simulink model "task2_3"  (R2023a)
settings: Solver=VariableStepAuto  StartTime=0.0  StopTime=10.0  RelTol=1e-3
settings Model: Creator=vasil  LastModifiedBy=vasil

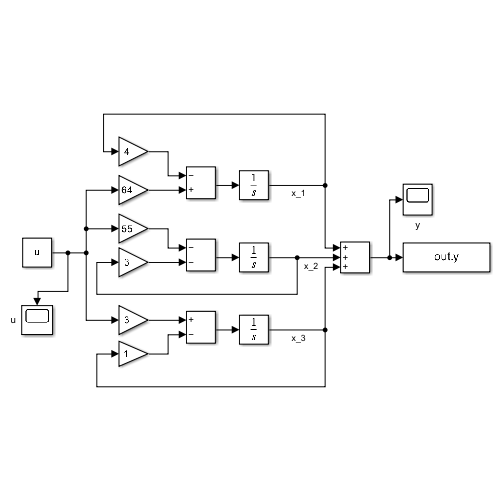
[thumbnail: Simulink's stored preview of the top-level diagram]
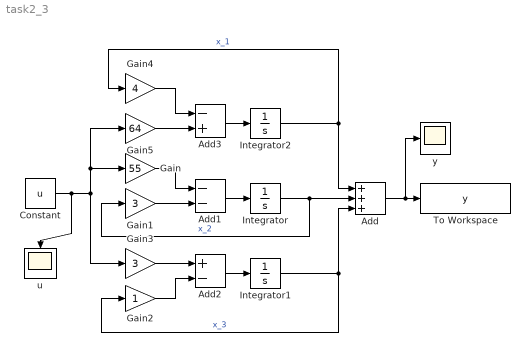
== system task2_3 ==
  Add : Sum  Inputs=+++
  Add1 : Sum  Inputs=--
  Add2 : Sum  Inputs=+-
  Add3 : Sum  Inputs=-+
  Constant : Constant  Value=u
  Gain : Gain  Gain=55
  Gain1 : Gain  Gain=3
  Gain2 : Gain
  Gain3 : Gain  Gain=3
  Gain4 : Gain  Gain=4
  Gain5 : Gain  Gain=64
  Integrator : Integrator
  Integrator1 : Integrator
  Integrator2 : Integrator
  To Workspace : ToWorkspace  VariableName=y  SaveFormat=Timeseries  SampleTime=-1
  u : Scope
  y : Scope
  wires:
  Add/1 -> y/1, To Workspace/1
  Integrator/1 -> Gain1/1, Add/2  "x_2"
  Integrator1/1 -> Gain2/1, Add/3  "x_3"
  Integrator2/1 -> Add/1, Gain4/1  "x_1"
  Add1/1 -> Integrator/1
  Add2/1 -> Integrator1/1
  Add3/1 -> Integrator2/1
  Gain/1 -> Add1/1
  Gain1/1 -> Add1/2
  Constant/1 -> u/1, Gain5/1, Gain/1, Gain3/1
  Gain3/1 -> Add2/1
  Gain2/1 -> Add2/2
  Gain5/1 -> Add3/2
  Gain4/1 -> Add3/1
